simulink subsystem "rw_to_accel"  (R2022b)
settings: Solver=VariableStepAuto  StartTime=0.0  StopTime=10.0  RelTol=1e-3
settings Model: Creator=Jon  LastModifiedBy=Jon
settings ModelReferenceCC: EnableRefExpFcnMdlSchedulingChecks=on

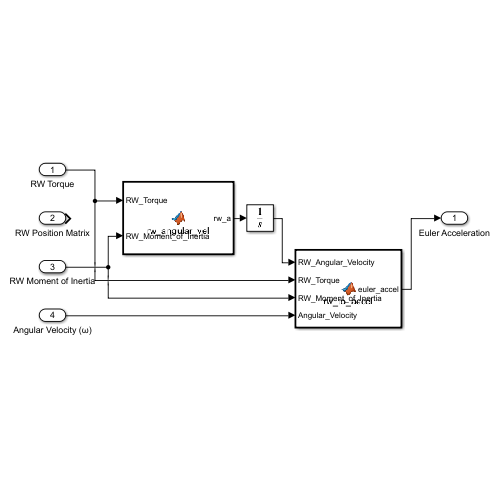
[thumbnail: Simulink's stored preview of the top-level diagram]
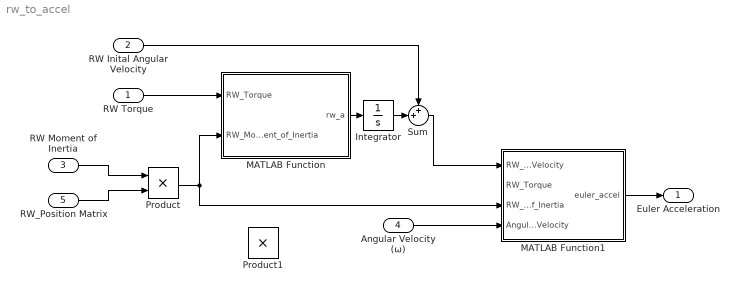
== system rw_to_accel ==
  RW Torque : Inport
  "RW Inital Angular Velocity " : Inport  Port=2
  RW Moment of Inertia : Inport  Port=3
  Angular Velocity (ω) : Inport  Port=4
  RW_Position Matrix : Inport  Port=5
  Integrator : Integrator
  MATLAB Function : MATLAB Function  TreatAsAtomicUnit=on
  MATLAB Function1 : MATLAB Function  TreatAsAtomicUnit=on
  Product : Product
  Product1 : Product
  Sum : Sum  Inputs=++|
  Euler Acceleration : Outport
  wires:
  MATLAB Function1/1(euler_accel) -> Euler Acceleration/1
  Angular Velocity (ω)/1 -> MATLAB Function1/4(Angular_Velocity)
  RW Torque/1 -> MATLAB Function/1(RW_Torque)
  MATLAB Function/1(rw_a) -> Integrator/1
  "RW Inital Angular Velocity "/1 -> Sum/1
  Integrator/1 -> Sum/2
  Sum/1 -> MATLAB Function1/1(RW_Angular_Velocity)
  RW Moment of Inertia/1 -> Product/1
  RW_Position Matrix/1 -> Product/2
  Product/1 -> MATLAB Function/2(RW_Moment_of_Inertia), MATLAB Function1/3(RW_Moment_of_Inertia)

== matlab function rw_to_accel/MATLAB Function1 ==
  data: RW_Angular_Velocity input; RW_Torque input; RW_Moment_of_Inertia input; Angular_Velocity input; euler_accel output
%% rw_to accel
% The function determines the euler acceleration of the satellite using the
% equation of motion from the system (desrcibed in the project notes)
% Inputs: RW_Angular_Velocity is a nx1 matrix, where n is the number of RWs,
% of the angular velocity of each RW. RW_Torque is a nx1 matrix of the
% torque applied to each RW. RW_Moment_of_Inertia is a 3xn matrix 
% representing the moment on intertia of the RWs (each RW has the same
% moment on interia, that is then applied to the sat. ref frame). 
% Angular_Velocity is an euler vector of the satellites angular velocity. 
% Ouput: euler_accel is an euler vector represetning the x, y and z 
% components of the angular acceleration.

function euler_accel = rw_to_accel(RW_Angular_Velocity,RW_Torque, RW_Moment_of_Inertia, Angular_Velocity)

ms2 = 3*0.1^2;
Ib = [5/6*ms2 0 0; 0 5/6*ms2 0; 0 0 1/6*ms2];
Ib_inv = inv(Ib);

w = Angular_Velocity;
wrw = RW_Angular_Velocity;
Irw = RW_Moment_of_Inertia;
Trw = RW_Torque;

term_one = cross(-Ib_inv*w, Ib*w);

[numRW, ~] = size(Trw);
term_sum = zeros(numRW,1);

%% TODO: fix this so that term_sum has vectors 
for i=1:numRW
    term_sum(i, :) = Trw(i) + cross(w,Irw(:,i)*wrw(i));
end

term_two = Ib_inv*sum(term_sum);

euler_accel = term_one - term_two;

end

== matlab function rw_to_accel/MATLAB Function ==
  data: RW_Torque input; rw_a output; RW_Moment_of_Inertia input
%% rw_angular_vel
% The function calculates the angular acceleration of each RW based
% on the applied torque, T, and moment on interita, I. (a = I-1 *T). 
% Inputs: RW_Torque is a nx1 matrix, where n is the number of RWs, of the
% torque applied to each RW. RW_Moment_of_Inertia is a 3xn matrix 
% representing the moment on intertia of the RWs (each RW has the same
% moment on interia) 
% Ouput: rw_a is nx1 matrix of the angular acceleration of each RW. (The
% acceleration is integrated outside of the function to determine the 
% angular velovity of each RW)

function rw_a = rw_angular_vel(RW_Torque, RW_Moment_of_Inertia)

% Irw_inv = inv(RW_Moment_of_Inertia);
Trw = RW_Torque;

[numRW, ~] = size(Trw);
rw_a = zeros(numRW,1);

for i=1:numRW
%     rw_a(i) = Irw_inv(:,i)*Trw(i);
    rw_a(i) = RW_Moment_of_Inertia(:,i)\Trw(i);
end

end
